simulink model "Three_PhaseRectifier_model"  (R2017a)
settings: Solver=VariableStepAuto  StartTime=0.0  StopTime=0.05  MaxStep=1e-4  RelTol=1e-3
libraries: powerlib x22
settings Model: Creator=sreer  LastModifiedBy=sreer

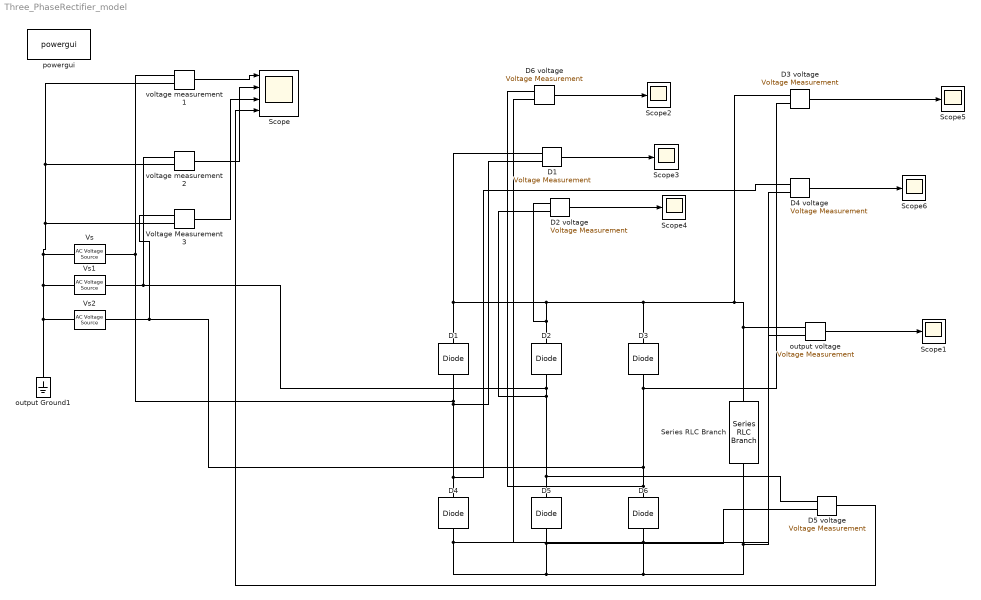
== system Three_PhaseRectifier_model ==
  D{1..6} (6 alike) : powerlib/Power Electronics/Diode  Ron=1e-3  Lon=0  Vf=0.7  IC=0  UseSnubber=off  Rs=1e6  Cs=inf  Measurements=off
  "D1 " : powerlib/Measurements/Voltage Measurement  PhasorSimulation=off  OutputType=Complex  PSBequivalent=0
  "D2 voltage " : powerlib/Measurements/Voltage Measurement  PhasorSimulation=off  OutputType=Complex  PSBequivalent=0
  D3 voltage : powerlib/Measurements/Voltage Measurement  PhasorSimulation=off  OutputType=Complex  PSBequivalent=0
  D4 voltage : powerlib/Measurements/Voltage Measurement  PhasorSimulation=off  OutputType=Complex  PSBequivalent=0
  D5 voltage : powerlib/Measurements/Voltage Measurement  PhasorSimulation=off  OutputType=Complex  PSBequivalent=0
  D6 voltage : powerlib/Measurements/Voltage Measurement  PhasorSimulation=off  OutputType=Complex  PSBequivalent=0
  Scope : Scope  NumInputPorts=4
  Scope{1..6} (6 alike) : Scope
  Series RLC Branch : powerlib/Elements/Series RLC Branch  LConnTagsString=__new0  RConnTagsString=__new0  BranchType=RL  Resistance=1  Inductance=1e-3  SetiL0=off  InitialCurrent=0  Capacitance=1e-6  Setx0=off  InitialVoltage=0  Measurements=None
  "Voltage Measurement3 " : powerlib/Measurements/Voltage Measurement  PhasorSimulation=off  OutputType=Complex  PSBequivalent=0
  Vs : powerlib/Electrical Sources/AC Voltage Source  Description=source block  Amplitude=120*sqrt(2)  Phase=90  Frequency=60  SampleTime=0  Measurements=Voltage  BusType=swing  Pref=10e3  Qref=0  Qmin=-inf  Qmax=+inf
      settings: AttributesFormatString=\n
  Vs1 : powerlib/Electrical Sources/AC Voltage Source  Description=source block  Amplitude=120*sqrt(2)  Phase=90+120  Frequency=60  SampleTime=0  Measurements=Voltage  BusType=swing  Pref=10e3  Qref=0  Qmin=-inf  Qmax=+inf
      settings: AttributesFormatString=\n
  Vs2 : powerlib/Electrical Sources/AC Voltage Source  Description=source block  Amplitude=120*sqrt(2)  Phase=90+240  Frequency=60  SampleTime=0  Measurements=Voltage  BusType=swing  Pref=10e3  Qref=0  Qmin=-inf  Qmax=+inf
      settings: AttributesFormatString=\n
  output Ground1 : powerlib/Elements/Ground  LConnTagsString=a
  output voltage : powerlib/Measurements/Voltage Measurement  PhasorSimulation=off  OutputType=Complex  PSBequivalent=0
  powergui : powerlib/powergui  Priority=1  SimulationMode=Continuous  SampleTime=50e-6  frequency=60  Iterations=50  frequencyindice=60  Pbase=100e6  ErrMax=1e-4  UnitsV=kV  UnitsW=MW  buscounter=0  FunctionMessages=off  echomessages=off  EnableUseOfTLC=off  CurrentSourceSwitches=off  DisableSnubberDevices=off  DisableRonSwitches=off  DisableVfSwitches=off  DisplayEquations=off  SolverType=Tustin/Backward Euler (TBE)  Interpol=off  ExternalGateDelay=off  methode=off  Ts=100  x0status=blocks  SPID=on  SwTol=0  HookPort=off  RestoreLinks=warning  ResistiveCurrentMeasurement=off  Frange=[0:2:500]  Ylog=off  Xlog=on  ShowGrid=off  save=off  variable=ZData  structure=0  ZoomFFT=off  StartTime=0.0  cycles=1  DisplayStyle=1  fundamental=60  FreqAxis=off  MaxFrequency=1000  frequencyindicesteady=1  RmsSteady=1  display=off
  "voltage measurement 1 " : powerlib/Measurements/Voltage Measurement  PhasorSimulation=off  OutputType=Complex  PSBequivalent=0
  "voltage measurement 2 " : powerlib/Measurements/Voltage Measurement  PhasorSimulation=off  OutputType=Complex  PSBequivalent=0
  wires:
  "voltage measurement 1 "/1 -> Scope/1
  "voltage measurement 2 "/1 -> Scope/2
  "Voltage Measurement3 "/1 -> Scope/3
  D5 voltage/1 -> Scope/4
  output voltage/1 -> Scope1/1
  D6 voltage/1 -> Scope2/1
  "D1 "/1 -> Scope3/1
  "D2 voltage "/1 -> Scope4/1
  D3 voltage/1 -> Scope5/1
  D4 voltage/1 -> Scope6/1
  connections:
  Vs/LConn1 -- "Voltage Measurement3 "/LConn2 -- "voltage measurement 2 "/LConn2 -- "voltage measurement 1 "/LConn2 -- Vs1/LConn1 -- Vs2/LConn1 -- output Ground1/LConn1
  D1/RConn1 -- "D1 "/LConn1 -- D3 voltage/LConn1 -- output voltage/LConn1 -- Series RLC Branch/LConn1 -- D3/RConn1 -- "D2 voltage "/LConn1 -- D2/RConn1
  D1/LConn1 -- "voltage measurement 1 "/LConn1 -- Vs/RConn1 -- "D1 "/LConn2 -- D4 voltage/LConn1 -- D4/RConn1
  D2/LConn1 -- "voltage measurement 2 "/LConn1 -- Vs1/RConn1 -- "D2 voltage "/LConn2 -- D5 voltage/LConn1 -- D5/RConn1
  D3/LConn1 -- D3 voltage/LConn2 -- "Voltage Measurement3 "/LConn1 -- Vs2/RConn1 -- D6 voltage/LConn1 -- D6/RConn1
  D4/LConn1 -- D4 voltage/LConn2 -- D5 voltage/LConn2 -- D5/LConn1 -- output voltage/LConn2 -- Series RLC Branch/RConn1 -- D6 voltage/LConn2 -- D6/LConn1
